simulink model "acc_with_sensor_copy"  (R2021b)
settings: Solver=FixedStepAuto  StartTime=0.0  StopTime=206  FixedStep=0.0005  RelTol=1e-3
InitFcn:
  | G=9.81;
  | m=1660;
  | rw=0.325;
  | Caf=74070;
  | Car=58525;
  | Iz=2778.5;
  | d = 1.502;
  | lf =1.1135;
  | lr =1.5065;
  | L = 2.62;
  | kph2mps=1/3.6;
values from neighbouring files (symbols this model uses):
  Leftdis_PV_switch = 2    [acc_plot_backup.m]
  s_path = [0 1.10508939428 2.2141958029 3.32141571172 4.42705301151 5.53154548532 6.63517443471 7.73808041313 8.84055018688 9.94289959674 11.0453539299 12.1480581097 ... (1001 elements, 1001x1)]    [200_100radius.mat]    (also in LV_Clothoid_S_Turn_path.mat = [0 0.966832089581 1.93621320584 2.90214024471 3.86476766313 ; NEDC_path.mat = [0 0.414605943146 0.832514087334 1.25401518562 1.68216660344; Straight_East_into_curve.mat = [0 1.65770560069 3.32192925577 4.98420060507 6.64484613518 8; acc_plot_backup.m = Station_HV_m)
  X_path = [0 1.10508939428 2.2141958029 3.32141571172 4.42705301151 5.53154548532 6.63517443471 7.73808041313 8.84055018688 9.94289959674 11.0453539299 12.1480581097 ... (1001 elements, 1001x1)]    [200_100radius.mat]    (also in LV_Clothoid_S_Turn_path.mat = [-10 -9.03316791042 -8.06378679416 -7.09785975529 -6.1352323; NEDC_path.mat = [0 0.414605943146 0.832514087334 1.25401518562 1.68216660344; Straight_East_into_curve.mat = [0 1.65770560069 3.32192925577 4.98420060507 6.64484613518 8; acc_plot_backup.m = X_HV_m)
  Y_path = [0 -1.70364610795e-18 -7.41532896709e-18 1.46822109542e-17 4.74557362791e-17 6.12980216762e-17 9.25043977736e-17 1.24088240159e-16 1.5099156923e-16 1.7058517853e-16 1.90629227614e-16 2.09673434424e-16 ... (1001 elements, 1001x1)]    [200_100radius.mat]    (also in LV_Clothoid_S_Turn_path.mat = [0 -8.46153035536e-19 5.07382551045e-18 2.07356032218e-17 3.; NEDC_path.mat = [0 -3.50680326162e-18 -2.14111304971e-18 3.38197671014e-18 3; Straight_East_into_curve.mat = [0 1.29197709199e-18 2.81882429322e-18 3.49020462564e-17 6.7; acc_plot_backup.m = Y_HV_m)
undefined symbols (not defined in the file or in its folder): C_TICK_TIME_S, Cut_in_Secenary_flg, ENUM_ACCSTATE_DISABLED, ENUM_ACCSTATE_OFF, ENUM_ACCSTATE_STANDBY, FALSE, KVDI_ACCLongPressTime_ms, KVDI_ACCMaxActSpeed_kph, KVDI_ACCSetSpdIntial_kph, KVDI_ACCSpdLargeChange_kph, KVDI_LongPressConTime_ms, ONE_FLOAT, ONE_INT, Path_selector, R, Rw, T, TRUE, UseTTC_switch, ZERO_FLOAT, ZERO_INT
libraries: simulink x15, dspstat3 x4, simulink_extras x2, Solver_SF x1
(part 8 of 8)

== matlab function acc_with_sensor_copy/QP_logitudinal1 ==
  data: u output; H input; f input; A_cons input; b input; u_old input
function u =QPhild(H,f,A_cons, b,u_old)
% E=H;
% F=f;
% M=A_cons;
% gamma=b;
% eta =x
% u_star = zeros(1);
% aa = ones(1);
[n1,m1]=size(A_cons);
% eta=H\f;
% kk=0;
% for i=1:n1
%     if (A_cons(i,:)*eta>b(i)) kk=kk+1;
%     else
%     kk=kk+0;
%     end
% end

% if (kk==0) return; end

P=A_cons*(H\A_cons');
d=(A_cons*(H\f)+b);
[n,m]=size(d);
x_ini=zeros(n,m);
lambda=x_ini;
al=10;

for km=1:25   %% P68
%     find the elements in the solution vector one by one
%     km could be larger if the Lagranger multiplier has a slow
%     convergence rate.
    lambda_p=lambda;
    for i=1:n
        w= P(i,:)*lambda-P(i,i)*lambda(i,1);
        w=w+d(i,1);
        la=-w/P(i,i);
        lambda(i,1)=max(0,la);
    end
    al=(lambda-lambda_p)'*(lambda-lambda_p);

    if (al<10e-8); break; end
end
eta=-H\f -H\A_cons'*lambda;

% eta=inv(H)*f;
% if isempty(eta)     %eta
%     [n1,m1]=size(A_cons_soft1);
%     eta1=-H\f;
%     kk=0;
%     for i=1:n1
%         if (A_cons_soft1(i,:)*eta1>b_soft1(i)) kk=kk+1;
%         else
%         kk=kk+0;
%         end
%     end
% 
%     if (kk==0) return; end
% 
%     P=A_cons_soft1*(H\A_cons_soft1');
%     d=(A_cons_soft1*(H\f)+b_soft1);
%     [n,m]=size(d);
%     x_ini=zeros(n,m);
%     lambda=x_ini;
%     al=10;
% 
%     for km=1:38
%         %find the elements in the solution vector one by one
%         % km could be larger if the Lagranger multiplier has a slow
%         % convergence rate.
%         lambda_p=lambda;
%         for i=1:n
%             w= P(i,:)*lambda-P(i,i)*lambda(i,1);
%             w=w+d(i,1);
%             la=-w/P(i,i);
%             lambda(i,1)=max(0,la);
%         end
%         al=(lambda-lambda_p)'*(lambda-lambda_p);
% 
%         if (al<10e-8); break; end
%     end
%     eta1=-H\f -H\A_cons_soft1'*lambda;
%     if isempty(eta1) %eta1
%         [n1,m1]=size(A_cons_soft2);
%         eta2=-H\f;
%         kk=0;
%         for i=1:n1
%             if (A_cons_soft2(i,:)*eta2>b_soft2(i)) kk=kk+1;
%             else
%             kk=kk+0;
%             end
%         end
% 
%         if (kk==0) return; end
% 
%         P=A_cons_soft2*(H\A_cons_soft2');
%         d=(A_cons_soft2*(H\f)+b_soft2);
%         [n,m]=size(d);
%         x_ini=zeros(n,m);
%         lambda=x_ini;
%         al=10;
% 
%         for km=1:38
%             %find the elements in the solution vector one by one
%             % km could be larger if the Lagranger multiplier has a slow
%             % convergence rate.
%             lambda_p=lambda;
%             for i=1:n
%                 w= P(i,:)*lambda-P(i,i)*lambda(i,1);
%                 w=w+d(i,1);
%                 la=-w/P(i,i);
%                 lambda(i,1)=max(0,la);
%             end
%             al=(lambda-lambda_p)'*(lambda-lambda_p);
% 
%             if (al<10e-8); break; end
%         end
%         eta2=-H\f -H\A_cons_soft2'*lambda;
%         u_star = eta2(1);
%     else
%         u_star = eta1(1);
%     end
% else
    aa = lambda(1);
    xk = eta(1);
    u=eta(1)+u_old;
end

== matlab function acc_with_sensor_copy/Kalman_Filter_LatSpd1 ==
  data: X_e output; X_e input; u input; Yaw_rate input; R input; Q input; y input; X_k output; F output; G output; G2 output; K output; M input; M2 output
function [X_e,X_k,F,G,G2,K,M2] = fcn(X_e,u,Yaw_rate,R,Q,y,M)
t= 0.1;

r_th= 0.015;

F = [1 Yaw_rate*t;
     -Yaw_rate*t 1];

G = [t 0;0 t];

G2 = [-X_e(2)*t -t 0;
       X_e(1)*t 0 -t];
X_k = F*X_e+G*u;
% X_k = F*X_e;
%%
Rn = R;
Qn = Q*[0.01 0 0;
       0 100 0;
       0 0 0.01];
H = [1 0];
P = M-M*H'*inv(H*M*H'+Rn)*H*M;
M2 = F*P*F'+G2*Qn*G2';
if abs(Yaw_rate)>=r_th
    K=P*H'*inv(Rn);
else
    K = zeros(2,1);
end
X_e=X_k+K*(y-H*X_k);
end

== stateflow chart acc_with_sensor_copy/ACC_Mode_Selector/Chart1 ==
  state ex_
    out=boolean(1);
  state Time
    en:
    TimeCLK=0
    du:
    TimeCLK=TimeCLK+0.1;
  state ex_1
    out=boolean(0);
  (default) -> ex_
  ex_1 -> ex_ : [flg==1]
  ex_ -> Time : [flg==0]
  Time -> ex_ [order 2] : [flg==1]
  Time -> ex_1 [order 1] : [TimeCLK>0.5]
  data: flg input; out output; count local; TimeCLK local

== matlab function acc_with_sensor_copy/MATLAB Function4 ==
  data: RR input; RX output; RD input; RY output
function [RX,RY] = fcn(RR,RD)
RX=RR*cosd(RD);
RY=RR*sind(RD);
end

== matlab function acc_with_sensor_copy/MATLAB Function6 ==
  data: Xf input; RR output; Yf input; Xh input; Yh input; RD output
function [RR,RD] = fcn(Xf,Yf,Xh,Yh)
RX=Xf-Xh;
RY=Yf-Yh;
if RX >= 0
    RR=sqrt(RX^2+RY^2);
    RD=atand(RY/RX);
else
    RR=sqrt(RX^2+RY^2);
    RD=atand(RY/RX)+180;
end
% if RD < -0.1
%     RD=RD+360;
% end
end

== matlab function acc_with_sensor_copy/LateralMotionKF1 ==
  data: T input; rk input; vxk input; delta input; Caf input; Car input; lf input; lr input; vyk1 output; mv input; vyk input; ayk output
function [vyk1,ayk] = fcn(T,rk,vxk,delta,Caf,Car,lf,lr,mv,vyk)
%%
if vxk >= 15/3.6
    ayk = -(Caf*( atan( (vyk+lf*rk)/vxk -delta) ) + Car*atan((vyk-lr*rk)/vxk))/mv;
else
    ayk = 0;
end

vyk1 = vyk-T*rk*vxk + T*ayk;
% vyk1 =T*ayk;

== matlab function acc_with_sensor_copy/Estimation_TTCx_PV1 ==
  data: R input; TTC1 output; V input; A input; TTC2 output
function [TTC1,TTC2] = TTCx(R,V,A)
TTCp1=10;
TTCp2=10;
if R < 0
    R=-R;
    V=-V;
    A=-A;
end
% if R > 7
%     R=R-7;
% else
%     R=0;
% end
if R <= 0.1 % buff
    TTC1=0;
else
    if abs(A) > 1 && (V^2-2*A*R)>0
        TTCp1=(-V+sqrt(V^2-2*A*R))/A;
        TTCp2=(-V-sqrt(V^2-2*A*R))/A;
        if TTCp1>0 && TTCp2 >0
            TTC1 =min(TTCp1,TTCp2);
        elseif TTCp1 >= 0
            TTC1=TTCp1;
        else
            TTC1=TTCp2;
        end
    else
    TTC1=-R/V;
    end
end

if TTC1 > 10 
    TTC1=10;
end
if TTC1 < 0 
    TTC1=10;
end

if R < 0.1
    TTC2=0;
else
    TTC2=-R/V;
end
if  TTC2 > 10
    TTC2=10;
end
if  TTC2 < 0
    TTC2=10;
end
end

== matlab function acc_with_sensor_copy/Subsystem5/MATLAB Function7 ==
  data: OnlyPV_signal input; RR_PV input; RR output; RV output; RA output; RR_APV input; RVx_PV input; RVx_APV input; RAx_PV input; RAx_APV input; RY_PV input; RY_APV input; RD_PV input; RD_APV input; trig output
function [RR,RV,RA,trig] = fcn(OnlyPV_signal,RR_PV,RR_APV,RVx_PV,RVx_APV,RAx_PV,RAx_APV,RY_PV,RY_APV,RD_PV,RD_APV)
if OnlyPV_signal==0
    if RR_APV < RR_PV && RY_APV-RY_PV <= 0.3 && RD_APV-RD_PV <= 5
        
        RR=RR_APV;
        RV=RVx_APV;
        RA=RAx_APV;
        trig=1;
    else
    
        RR=RR_PV;
        RV=RVx_PV;
        RA=RAx_PV;
        trig=0;
    end
else
    RR=RR_PV;
    RV=RVx_PV;
    RA=RAx_PV;
    trig=0;
end

end

== matlab function acc_with_sensor_copy/Estimation_TTCx_PV2 ==
  data: R input; TTC1 output; V input; A input; TTC2 output
function [TTC1,TTC2] = TTCx(R,V,A)
up_bound=10;
TTCp1=up_bound;
TTCp2=up_bound;
if R < 0
    R=-R;
    V=-V;
    A=-A;
end
% if R > 7
%     R=R-7;
% else
%     R=0;
% end
if R <= 0.1 % buff
    TTC1=0;
else
    if abs(A) > 1 && (V^2-2*A*R)>0
        TTCp1=(-V+sqrt(V^2-2*A*R))/A;
        TTCp2=(-V-sqrt(V^2-2*A*R))/A;
        if TTCp1>0 && TTCp2 >0
            TTC1 =min(TTCp1,TTCp2);
        elseif TTCp1 >= 0
            TTC1=TTCp1;
        else
            TTC1=TTCp2;
        end
    else
    TTC1=-R/V;
    end
end

if TTC1 > up_bound
    TTC1=up_bound;
end
if TTC1 < 0 
    TTC1=up_bound;
end

if R < 0.1
    TTC2=0;
else
    TTC2=-R/V;
end
if  TTC2 > up_bound
    TTC2=up_bound;
end
if  TTC2 < 0
    TTC2=up_bound;
end
end
